simulink model "nonlinear_ode_modeimp"  (R2019b)
settings: Solver=ode45  StartTime=1.0  StopTime=5.0  MaxStep=0.01  RelTol=1e-3
settings Model: Creator=andrey  LastModifiedBy=Roman
settings DebuggingCC: UnconnectedInputMsg=none  UnconnectedOutputMsg=none  UnconnectedLineMsg=none
settings ModelReferenceCC: EnableRefExpFcnMdlSchedulingChecks=off
settings RTWCC: Description=Generic Real-Time Target

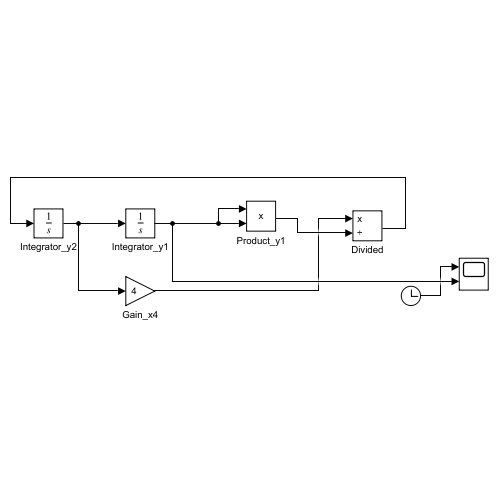
[thumbnail: Simulink's stored preview of the top-level diagram]
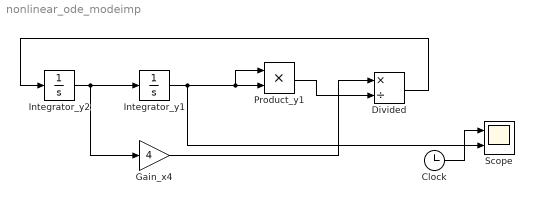
== system nonlinear_ode_modeimp ==
  Clock : Clock
  Divided : Product  Inputs=*/
  Gain_x4 : Gain  Gain=4
  Integrator_y1 : Integrator  InitialCondition=1
  Integrator_y2 : Integrator  InitialCondition=-4
  Product_y1 : Product
  Scope : Scope  NumInputPorts=2
  wires:
  Integrator_y2/1 -> Gain_x4/1, Integrator_y1/1
  Integrator_y1/1 -> Scope/2, Product_y1/1, Product_y1/2
  Gain_x4/1 -> Divided/1
  Product_y1/1 -> Divided/2
  Divided/1 -> Integrator_y2/1
  Clock/1 -> Scope/1
